simulink model "model"  (R2014a)
settings: Solver=FixedStepDiscrete  StartTime=0.0  StopTime=N/Fs  RelTol=1e-3
model workspace: external: MAT-File (data not in the file)
values from neighbouring files (symbols this model uses):
  Fs = sscanf(ECG.SamplingFrequency, '    [simulate.m]
  J = round(log2(Fs))    [init_model.m]    (also in simulate.m = ecg_detect_jay_points(X, Fs, h+1))
  N = length(ECG)    [init_model.m]    (also in simulate.m = length(X))
  wdelay = round(2.^((J:-1:1)-1)*(d0+d1)-d0)    [init_model.m]
libraries: dspsigops x8, simulink x8, dspsnks4 x3, dspmlti4 x2, dspsrcs4 x1, dspstat3 x1
settings Model: ExtModeTrigMode=oneshot  ExtModeArmWhenConnect=off  Creator=The MathWorks Inc.  LastModifiedBy=Diego Sogari
settings DataIOCC: LimitDataPoints=off  SignalLoggingSaveFormat=ModelDataLogs  SaveOutput=off  SaveTime=off  SignalLoggingName=sigsOut
settings OptimizationCC: BlockReduction=off  BooleanDataType=off  ExpressionDepthLimit=2147483647  InitFltsAndDblsToZero=on  EfficientMapNaN2IntZero=off
settings DebuggingCC: SaveWithParameterizedLinksMsg=none  UnderspecifiedInitializationDetection=Classic  SignalResolutionControl=TryResolveAllWithWarning  SolverPrmCheckMsg=none  MultiTaskDSMMsg=warning  MultiTaskCondExecSysMsg=none  IntegerOverflowMsg=none  FcnCallInpInsideContextMsg=UseLocalSettings  StateNameClashWarn=warning
settings HardwareCC: TargetUnknown=on
settings RTWCC: IncludeERTFirstTime=on
settings GRTTargetCC: TargetFcnLib=ansi_tfl_tmw.mat  CombineOutputUpdateFcns=off  GRTInterface=on

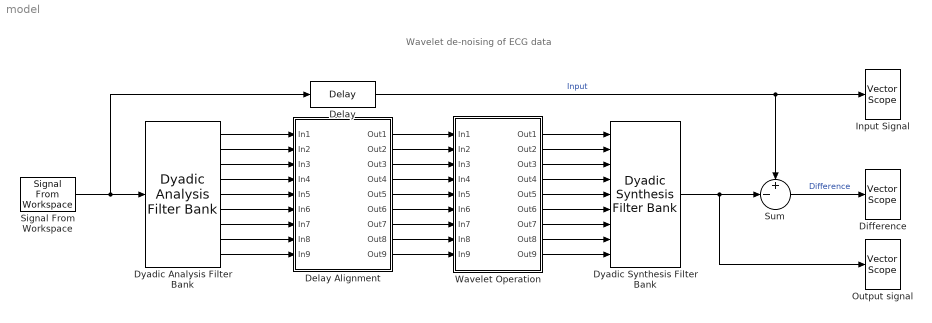
== system model ==
  note: Wavelet de-noising of ECG data
  Delay : dspsigops/Delay  InputProcessing=Columns as channels (frame based)  dly_unit=Samples  delay=wdelay0  ic_detail=on  dif_ic_for_ch=off  dif_ic_for_dly=off  ic=0  reset_popup=None
  Delay Alignment : Subsystem
  Difference : dspsnks4/Vector Scope  ScopeProperties=on  Domain=Time  HorizSpan=15  DisplayProperties=off  AxisGrid=on  Memory=off  FrameNumber=on  AxisLegend=off  AxisZoom=off  OpenScopeAtSimStart=on  OpenScopeImmediately=off  FigPos=[484 228 430 200]  AxisProperties=off  XUnits=Hertz  XRange=[0...Fs/2]  InheritXIncr=on  XIncr=1  XLabel=Samples  XLimit=Auto  XMin=0  XMax=N/Fs  XStart=0  YUnits=dB  YLabel=Amplitude  LineProperties=off  XAxisParamsVer=6.9
      settings: YMin=-3e-15  YMax=2e-15
  Dyadic Analysis Filter Bank : dspmlti4/Dyadic Analysis Filter Bank  Wname=User-defined  OrdRec_ordDec=[3 / 5]  Order=4  LPF=lod  HPF=hid  NumLevels=J  tree=Asymmetric  Output=Multiple ports
  Dyadic Synthesis Filter Bank : dspmlti4/Dyadic Synthesis Filter Bank  Wname=User-defined  OrdRec_ordDec=[3 / 5]  Order=4  LPF=lor  HPF=hir  NumLevels=J  tree=Asymmetric  Input=Multiple ports
  Input Signal : dspsnks4/Vector Scope  ScopeProperties=on  Domain=Time  HorizSpan=15  DisplayProperties=off  AxisGrid=on  Memory=off  FrameNumber=on  AxisLegend=off  AxisZoom=off  OpenScopeAtSimStart=on  OpenScopeImmediately=off  FigPos=[46 513 430 200]  AxisProperties=off  XUnits=Hertz  XRange=[0...Fs/2]  InheritXIncr=on  XIncr=1  XLabel=Samples  XLimit=Auto  XMin=0  XMax=N/Fs  XStart=0  YUnits=dB  YLabel=Amplitude  LineProperties=off  XAxisParamsVer=6.9
      settings: YMin=-2  YMax=3
  Output signal : dspsnks4/Vector Scope  ScopeProperties=on  Domain=Time  HorizSpan=15  DisplayProperties=off  AxisGrid=on  Memory=off  FrameNumber=on  AxisLegend=off  AxisZoom=off  OpenScopeAtSimStart=on  OpenScopeImmediately=off  FigPos=[484 512 430 200]  AxisProperties=off  XUnits=Hertz  XRange=[0...Fs/2]  InheritXIncr=on  XIncr=1  XLabel=Samples  XLimit=Auto  XMin=0  XMax=N/Fs  XStart=0  YUnits=dB  YLabel=Amplitude  LineProperties=off  XAxisParamsVer=6.9
      settings: YMin=-2  YMax=3
  Signal From Workspace : dspsrcs4/Signal From Workspace  X=ECG  Ts=1/Fs  nsamps=2^J  OutputAfterFinalValue=Setting to zero  ignoreOrWarnInputAndFrameLengths=off
  Sum : Sum  Inputs=+-|  SaturateOnIntegerOverflow=on  InputSameDT=on  OutDataTypeStr=Inherit: Same as first input
  Wavelet Operation : Subsystem  mask{baseline=on, noise=off, bias=0}
      mask prompts: baseline "Remove baseline"; noise "Remove noise"
      mask init:
      | if baseline || noise
      |     str = 'Denoise';
      | else
      |     str = 'Reconstruct';
      | end
      mask Callback baseline:
      | params = get_param(gcb, 'MaskValues');
      | set_param(gcb,'MaskEnables',{'on','on',params{1}});
      mask Display: disp(str)
  wires:
  Delay/1 -> Input Signal/1, Sum/1  "Input"
  Sum/1 -> Difference/1  "Difference"
  Signal From Workspace/1 -> Delay/1, Dyadic Analysis Filter Bank/1
  Dyadic Synthesis Filter Bank/1 -> Sum/2, Output signal/1
  Dyadic Analysis Filter Bank/1 -> Delay Alignment/1(In1)
  Dyadic Analysis Filter Bank/8 -> Delay Alignment/8(In8)
  Dyadic Analysis Filter Bank/9 -> Delay Alignment/9(In9)
  Dyadic Analysis Filter Bank/4 -> Delay Alignment/4(In4)
  Dyadic Analysis Filter Bank/6 -> Delay Alignment/6(In6)
  Dyadic Analysis Filter Bank/5 -> Delay Alignment/5(In5)
  Dyadic Analysis Filter Bank/7 -> Delay Alignment/7(In7)
  Dyadic Analysis Filter Bank/2 -> Delay Alignment/2(In2)
  Dyadic Analysis Filter Bank/3 -> Delay Alignment/3(In3)
  Delay Alignment/7(Out7) -> Wavelet Operation/7(In7)
  Delay Alignment/8(Out8) -> Wavelet Operation/8(In8)
  Delay Alignment/5(Out5) -> Wavelet Operation/5(In5)
  Delay Alignment/6(Out6) -> Wavelet Operation/6(In6)
  Delay Alignment/9(Out9) -> Wavelet Operation/9(In9)
  Delay Alignment/1(Out1) -> Wavelet Operation/1(In1)
  Delay Alignment/2(Out2) -> Wavelet Operation/2(In2)
  Delay Alignment/4(Out4) -> Wavelet Operation/4(In4)
  Delay Alignment/3(Out3) -> Wavelet Operation/3(In3)
  Wavelet Operation/2(Out2) -> Dyadic Synthesis Filter Bank/2
  Wavelet Operation/3(Out3) -> Dyadic Synthesis Filter Bank/3
  Wavelet Operation/4(Out4) -> Dyadic Synthesis Filter Bank/4
  Wavelet Operation/5(Out5) -> Dyadic Synthesis Filter Bank/5
  Wavelet Operation/6(Out6) -> Dyadic Synthesis Filter Bank/6
  Wavelet Operation/1(Out1) -> Dyadic Synthesis Filter Bank/1
  Wavelet Operation/7(Out7) -> Dyadic Synthesis Filter Bank/7
  Wavelet Operation/9(Out9) -> Dyadic Synthesis Filter Bank/9
  Wavelet Operation/8(Out8) -> Dyadic Synthesis Filter Bank/8

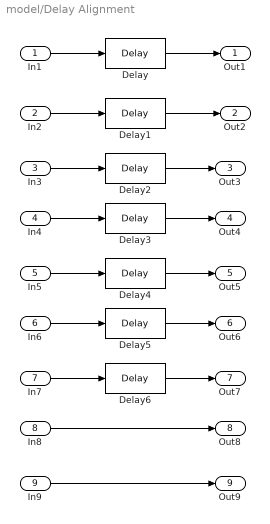
== system model/Delay Alignment ==
  In1 : Inport
  In2 : Inport  Port=2
  In3 : Inport  Port=3
  In4 : Inport  Port=4
  In5 : Inport  Port=5
  In6 : Inport  Port=6
  In7 : Inport  Port=7
  In8 : Inport  Port=8
  In9 : Inport  Port=9
  Delay : dspsigops/Delay  InputProcessing=Columns as channels (frame based)  dly_unit=Samples  delay=wdelay(1)  ic_detail=on  dif_ic_for_ch=off  dif_ic_for_dly=off  ic=0  reset_popup=None
  Delay1 : dspsigops/Delay  InputProcessing=Columns as channels (frame based)  dly_unit=Samples  delay=wdelay(2)  ic_detail=on  dif_ic_for_ch=off  dif_ic_for_dly=off  ic=0  reset_popup=None
  Delay2 : dspsigops/Delay  InputProcessing=Columns as channels (frame based)  dly_unit=Samples  delay=wdelay(3)  ic_detail=on  dif_ic_for_ch=off  dif_ic_for_dly=off  ic=0  reset_popup=None
  Delay3 : dspsigops/Delay  InputProcessing=Columns as channels (frame based)  dly_unit=Samples  delay=wdelay(4)  ic_detail=on  dif_ic_for_ch=off  dif_ic_for_dly=off  ic=0  reset_popup=None
  Delay4 : dspsigops/Delay  InputProcessing=Columns as channels (frame based)  dly_unit=Samples  delay=wdelay(5)  ic_detail=on  dif_ic_for_ch=off  dif_ic_for_dly=off  ic=0  reset_popup=None
  Delay5 : dspsigops/Delay  InputProcessing=Columns as channels (frame based)  dly_unit=Samples  delay=wdelay(6)  ic_detail=on  dif_ic_for_ch=off  dif_ic_for_dly=off  ic=0  reset_popup=None
  Delay6 : dspsigops/Delay  InputProcessing=Columns as channels (frame based)  dly_unit=Samples  delay=wdelay(7)  ic_detail=on  dif_ic_for_ch=off  dif_ic_for_dly=off  ic=0  reset_popup=None
  Out1 : Outport
  Out2 : Outport  Port=2
  Out3 : Outport  Port=3
  Out4 : Outport  Port=4
  Out5 : Outport  Port=5
  Out6 : Outport  Port=6
  Out7 : Outport  Port=7
  Out8 : Outport  Port=8
  Out9 : Outport  Port=9
  wires:
  In1/1 -> Delay/1
  Delay/1 -> Out1/1
  In5/1 -> Delay4/1
  Delay4/1 -> Out5/1
  In4/1 -> Delay3/1
  Delay3/1 -> Out4/1
  In3/1 -> Delay2/1
  Delay2/1 -> Out3/1
  In2/1 -> Delay1/1
  Delay1/1 -> Out2/1
  In8/1 -> Out8/1
  In9/1 -> Out9/1
  In6/1 -> Delay5/1
  In7/1 -> Delay6/1
  Delay6/1 -> Out7/1
  Delay5/1 -> Out6/1

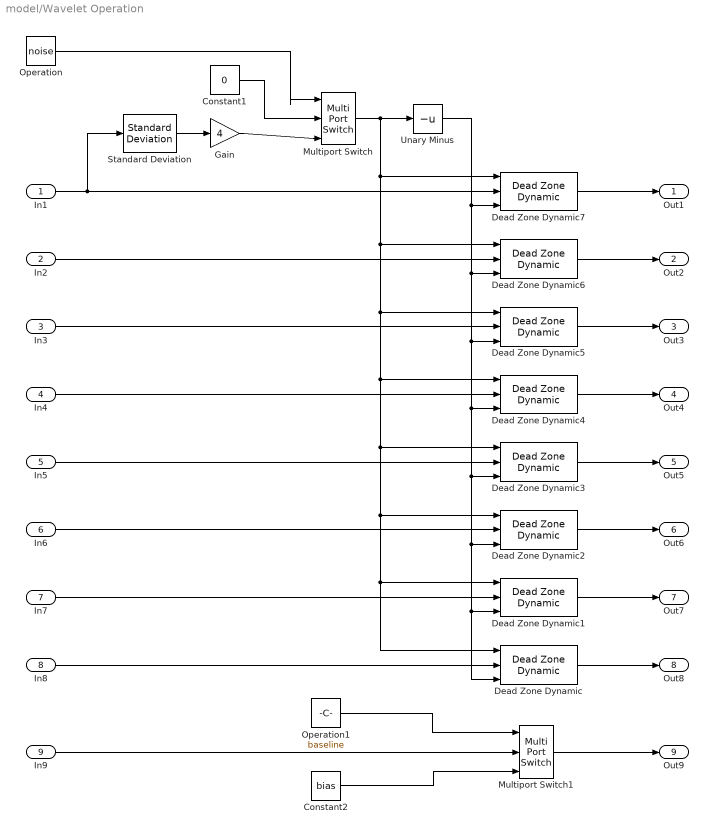
== system model/Wavelet Operation ==
  In1 : Inport
  In2 : Inport  Port=2
  In3 : Inport  Port=3
  In4 : Inport  Port=4
  In5 : Inport  Port=5
  In6 : Inport  Port=6
  In7 : Inport  Port=7
  In8 : Inport  Port=8
  In9 : Inport  Port=9
  Constant1 : Constant  Value=0
  Constant2 : Constant  Value=bias
  Dead Zone Dynamic{,1..7} (8 alike) : simulink/Discontinuities/Dead Zone Dynamic
  Gain : Gain  Gain=4
  Multiport Switch : MultiPortSwitch  DataPortOrder=Zero-based contiguous  Inputs=2
  Multiport Switch1 : MultiPortSwitch  DataPortOrder=Zero-based contiguous  Inputs=2
  Operation : Constant  Value=noise
  Operation1 : Constant  Value=baseline
  Standard Deviation : dspstat3/Standard Deviation  run=off  reset_popup=None  InputProcessing=Columns as channels (frame based)  directionMode=Each column  dimension=1  treatSBRowAsCol=on  roiEnable=off  roiType=Rectangles  roiPortion=Entire ROI  roiOutput=Individual statistics for each ROI  roiFlag=off
  Unary Minus : UnaryMinus
  Out1 : Outport
  Out2 : Outport  Port=2
  Out3 : Outport  Port=3
  Out4 : Outport  Port=4
  Out5 : Outport  Port=5
  Out6 : Outport  Port=6
  Out7 : Outport  Port=7
  Out8 : Outport  Port=8
  Out9 : Outport  Port=9
  wires:
  Dead Zone Dynamic4/1 -> Out4/1
  Dead Zone Dynamic6/1 -> Out2/1
  Dead Zone Dynamic5/1 -> Out3/1
  Dead Zone Dynamic2/1 -> Out6/1
  Unary Minus/1 -> Dead Zone Dynamic/3, Dead Zone Dynamic1/3, Dead Zone Dynamic2/3, Dead Zone Dynamic3/3, Dead Zone Dynamic4/3, Dead Zone Dynamic5/3, Dead Zone Dynamic6/3, Dead Zone Dynamic7/3
  Dead Zone Dynamic3/1 -> Out5/1
  Multiport Switch/1 -> Dead Zone Dynamic/1, Dead Zone Dynamic1/1, Dead Zone Dynamic2/1, Dead Zone Dynamic3/1, Dead Zone Dynamic4/1, Dead Zone Dynamic5/1, Dead Zone Dynamic6/1, Dead Zone Dynamic7/1, Unary Minus/1
  Dead Zone Dynamic7/1 -> Out1/1
  In2/1 -> Dead Zone Dynamic6/2
  In3/1 -> Dead Zone Dynamic5/2
  In4/1 -> Dead Zone Dynamic4/2
  In5/1 -> Dead Zone Dynamic3/2
  In6/1 -> Dead Zone Dynamic2/2
  Standard Deviation/1 -> Gain/1
  In1/1 -> Dead Zone Dynamic7/2, Standard Deviation/1
  Gain/1 -> Multiport Switch/3
  Operation/1 -> Multiport Switch/1
  Constant1/1 -> Multiport Switch/2
  Constant2/1 -> Multiport Switch1/3
  Operation1/1 -> Multiport Switch1/1
  Multiport Switch1/1 -> Out9/1
  Dead Zone Dynamic/1 -> Out8/1
  In7/1 -> Dead Zone Dynamic1/2
  In8/1 -> Dead Zone Dynamic/2
  In9/1 -> Multiport Switch1/2
  Dead Zone Dynamic1/1 -> Out7/1
